simulink model "mathtest"  (R2022b)
settings: Solver=FixedStepAuto  StartTime=0.0  StopTime=10.0  FixedStep=.01  RelTol=1e-3
settings Model: Creator=hollis  LastModifiedBy=hollis

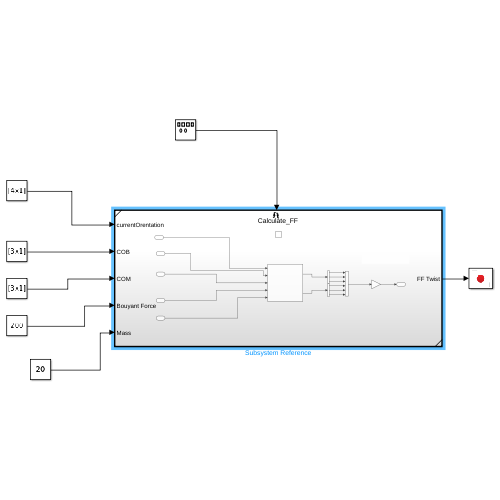
[thumbnail: Simulink's stored preview of the top-level diagram]
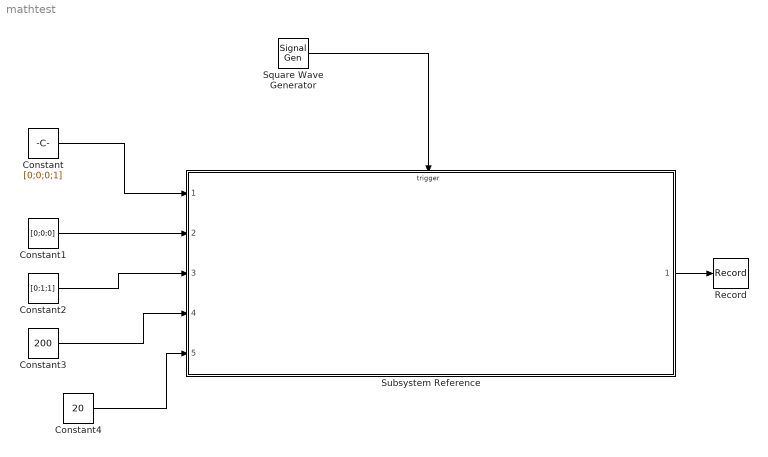
== system mathtest ==
  Constant : Constant  Value=[0;0;0;1]
  Constant1 : Constant  Value=[0;0;0]
  Constant2 : Constant  Value=[0;1;1]
  Constant3 : Constant  Value=200
  Constant4 : Constant  Value=20
  Record : Record  FileSettingsInternal="{\"entries\":[{\"content\":{\"excelSettings\":{\"content\":{},\"type\":\"Streamout.ExcelSettings\"}},\"type\":\"Streamout.FileSettingStorage\",\"uuid\":\"e5c24055-3009-4615-bb81-fb81a7f47fd5\"}],\"packageUris\":[\"http://schema.mathworks.com/mf0/streamout_blocks/R2020a\"],\"version\":\"1.0\"}"  Layout=[1 1]  SignalsInternal="{\"entries\":[{\"content\":{\"signals\":[{\"content\":{\"blockPath\":[\"mathtest/Record\"],\"channel\":[],\"dimensions\":[6],\"domain\":\"mathtest/Record\",\"hasChildren\":true,\"lineColor\":\"#ff6929\",\"plots\":[],\"port\":1,\"sid\":[\"\"],\"signalID\":601,\"signalName\":\"Subsystem Reference\"},\"type\":\"RecordBlkView.Signal\",\"uuid\":\"635a73b0-1371-42c7-88cb-9ccc1e8014a1\"},{\"content\":{\"blockPath\":[\"mathtest/Record\"],\"channel\":[1],\"dimensions\":[6],\"domain\":\"mathtest/Record\",\"lineColor\":\"#7e2f8e\",\"parentID\":601,\"plots\":[1],\"port\":1,\"sid\":[\"\"],\"signalID\":602,\"signalName\":\"Subsystem Reference\"},\"type\":\"RecordBlkView.Signal\",\"uuid\":\"931e2922-15d4-4d8e-8ff9-d90f023a7ce6\"},{\"content\":{\"blockPath\":[\"mathtest/Record\"],\"channel\":[2],\"dimensions\":[6],\"domain\":\"mathtest/Record\",\"lineColor\":\"#77ac30\",\"parentID\":601,\"plots\":[1],\"port\":1,\"sid\":[\"\"],\"signalID\":608,\"signalName\":\"Subsystem Reference\"},\"type\":\"RecordBlkView.Signal\",\"uuid\":\"66f64cbe-f510-431a-b355-761d7fe95ae9\"},{\"content\":{\"blockPath\":[\"mathtest/Record\"],\"channel\":[3],\"dimensions\":[6],\"domain\":\"mathtest/Record\",\"lineColor\":\"#4dbeee\",\"parentID\":601,\"plots\":[1],\"port\":1,\"sid\":[\"\"],\"signalID\":609,\"signalName\":\"Subsystem Reference\"},\"type\":\"RecordBlkView.Signal\",\"uuid\":\"760ac3f1-345b-438a-a729-4a0e12021693\"},{\"content\":{\"blockPath\":[\"mathtest/Record\"],\"channel\":[4],\"dimensions\":[6],\"domain\":\"mathtest/Record\",\"lineColor\":\"#a2142f\",\"parentID\":601,\"plots\":[1],\"port\":1,\"sid\":[\"\"],\"signalID\":610,\"signalName\":\"Subsystem Reference\"},\"type\":\"RecordBlkView.Signal\",\"uuid\":\"030b0984-0522-40f6-aa7b-e17e7cec6f16\"},{\"content\":{\"blockPath\":[\"mathtest/Record\"],\"channel\":[5],\"dimensions\":[6],\"domain\":\"mathtest/Record\",\"lineColor\":\"#139fff\",\"parentID\":601,\"plots\":[1],\"port\":1,\"sid\":[\"\"],\"signalID\":611,\"signalName\":\"Subsystem Reference\"},\"type\":\"RecordBlkView.Signal\",\"uuid\":\"f3725985-adbc-4304-a343-84087c73f132\"},{\"content\":{\"blockPath\":[\"mathtest/Record\"],\"channel\":[6],\"dimensions\":[6],\"domain\":\"mathtest/Record\",\"lineColor\":\"#ff6929\",\"parentID\":601,\"plots\":[1],\"port\":1,\"sid\":[\"\"],\"signalID\":612,\"signalName\":\"Subsystem Reference\"},\"type\":\"RecordBlkView.Signal\",\"uuid\":\"876e203a-2513-40d3-bdf1-5561faf0eb4b\"}]},\"type\":\"RecordBlkView.InputSignals\",\"uuid\":\"6725a502-8fb9-474e-8460-7c9a1f4f4b82\"}],\"packageUris\":[\"http://schema.mathworks.com/mf0/streamout_blocks/R2020a\"],\"version\":\"1.0\"}"  VisualizationBindings="{\"sparklinesplugin\":{\"info\":[{\"bindingParametersList\":[],\"subplotID\":1}]}}"
  Square Wave Generator : SignalGenerator  WaveForm=square  Frequency=100
  Subsystem Reference : Subsystem  ReferencedSubsystem=Calculate_FF
  wires:
  Constant/1 -> Subsystem Reference/1
  Constant1/1 -> Subsystem Reference/2
  Constant2/1 -> Subsystem Reference/3
  Constant3/1 -> Subsystem Reference/4
  Constant4/1 -> Subsystem Reference/5
  Subsystem Reference/1 -> Record/1
  Square Wave Generator/1 -> Subsystem Reference/Trigger
